simulink model "DuctedFanMolell_V1"  (R2021b)
settings: Solver=VariableStepAuto  StartTime=0.0  StopTime=50.2  MaxStep=0.01  RelTol=1e-3
undefined symbols (not defined in the file or in its folder): SimParam
settings Model: PacingRate=1.300000  VariantFading=off  Creator=tim  LastModifiedBy=tim

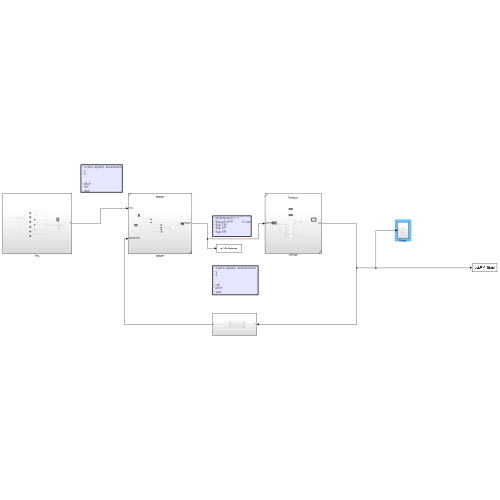
[thumbnail: Simulink's stored preview of the top-level diagram]
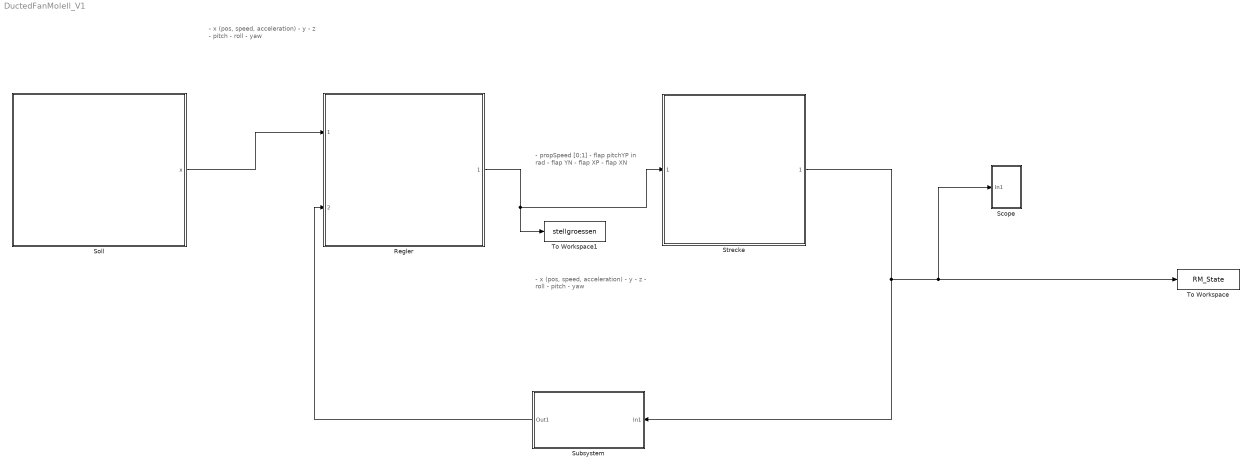
== system DuctedFanMolell_V1 ==
  note: - x (pos, speed, acceleration)
      | - y
      | - z
      |
      |
      | - roll
      | - pitch
      | - yaw
  note: - x (pos, speed, acceleration)
      | - y
      | - z
      |
      |
      | - pitch
      | - roll
      | - yaw
  note: - propSpeed [0;1]
      | - flap pitchYP          in rad
      | - flap YN
      | - flap XP
      | - flap XN
  Regler : Subsystem  VariantControl=Choice  ReferencedSubsystem=Regler
  Scope : Subsystem
  Soll : Subsystem
  Strecke : Subsystem  ReferencedSubsystem=Strecke
  Subsystem : Subsystem
      settings: PortSchema="{\"entries\":[{\"content\":{\"sides\":[{\"content\":{\"connectorIds\":[\"Out1\"]},\"type\":\"ConnectorPlacement.EquallySpacedRectSide\",\"uuid\":\"0b6b1713-0599-4a2b-a6b8-17ca65ceb7bc\"},{\"content\":{\"connectorIds\":[\"In1\"],\"side\":\"RIGHT\"},\"type\":\"ConnectorPlacement.EquallySpacedRectSide\",\"uuid\":\"89969f44-fab1-4e90-b2ff-0e3a2cc6e655\"},{\"content\":{\"connectorIds\":[],\"side\":\"TOP\"},\"type\":\"ConnectorPlacement.EquallySpacedRectSide\",\"uuid\":\"aad73966-e619-409d-ac58-96523cc99cf8\"}]},\"type\":\"ConnectorPlacement.EquallySpacedConnector\",\"uuid\":\"181e3664-8f4e-4946-ae8e-84605a680910\"}],\"packageUris\":[\"http://schema.mathworks.com/mf0/Connector/R2020b\"],\"version\":\"1.0\"}"
  To Workspace : ToWorkspace  VariableName=RM_State  SaveFormat=Timeseries  SampleTime=-1
  To Workspace1 : ToWorkspace  VariableName=stellgroessen  SaveFormat=Timeseries  SampleTime=-1
  wires:
  Soll/1(x) -> Regler/1
  Strecke/1 -> Subsystem/1(In1), Scope/1(In1), To Workspace/1
  Regler/1 -> To Workspace1/1, Strecke/1
  Subsystem/1(Out1) -> Regler/2

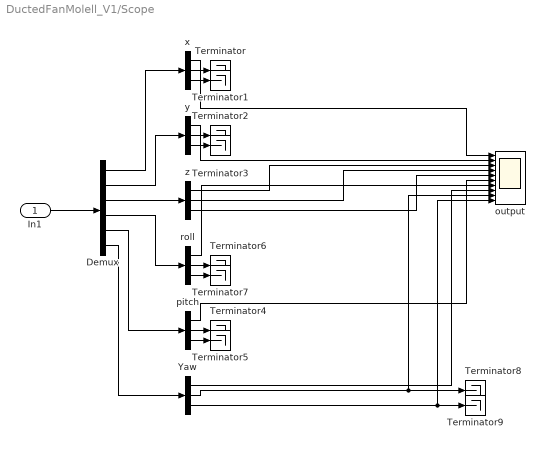
== system DuctedFanMolell_V1/Scope ==
  In1 : Inport
  Demux : Demux  Outputs=[3 3 3 3 3 3]
  Terminator{,1..9} (10 alike) : Terminator
  Yaw : Demux  Outputs=3
  output : Scope  NumInputPorts=10
  pitch : Demux  Outputs=3
  roll : Demux  Outputs=3
  x : Demux  Outputs=3
  y : Demux  Outputs=3
  z : Demux  Outputs=3
  wires:
  Demux/4 -> roll/1
  y/1 -> output/2
  y/2 -> Terminator2/1
  z/3 -> output/5
  Demux/1 -> x/1
  z/2 -> output/4
  roll/2 -> Terminator6/1
  Demux/6 -> Yaw/1
  pitch/3 -> Terminator5/1
  Yaw/2 -> output/9, Terminator8/1
  x/3 -> Terminator1/1
  x/1 -> output/1
  pitch/2 -> Terminator4/1
  Demux/3 -> z/1
  y/3 -> Terminator3/1
  Yaw/3 -> output/10, Terminator9/1
  roll/3 -> Terminator7/1
  pitch/1 -> output/6
  Yaw/1 -> output/8
  In1/1 -> Demux/1
  roll/1 -> output/7
  z/1 -> output/3
  Demux/5 -> pitch/1
  x/2 -> Terminator/1
  Demux/2 -> y/1

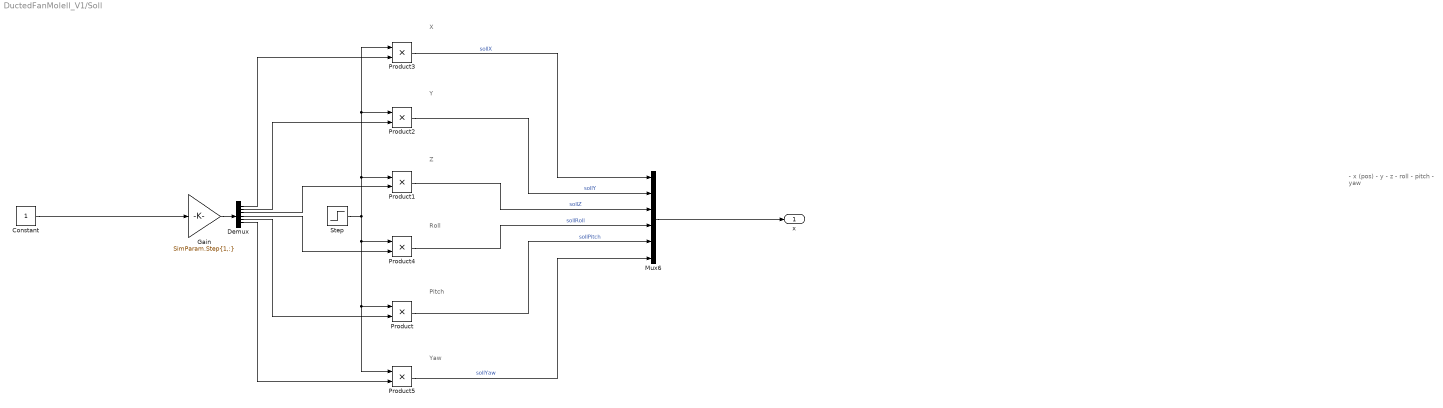
== system DuctedFanMolell_V1/Soll ==
  note: Y
  note: - x (pos)
      | - y
      | - z
      |
      |
      | - roll
      | - pitch
      | - yaw
  note: X
  note: Z
  note: Pitch
  note: Roll
  note: Yaw
  Constant : Constant
  Demux : Demux  Outputs=6
  Gain : Gain  Gain=SimParam.Step{1,:}
  Mux6 : Mux  Inputs=6
  Product{,1..5} (6 alike) : Product
  Step : Step  SampleTime=0
  x : Outport
  wires:
  Product3/1 -> Mux6/1  "sollX"
  Product2/1 -> Mux6/2  "sollY"
  Product1/1 -> Mux6/3  "sollZ"
  Product4/1 -> Mux6/4  "sollRoll"
  Product5/1 -> Mux6/6  "sollYaw"
  Product/1 -> Mux6/5  "sollPitch"
  Mux6/1 -> x/1
  Demux/5 -> Product/2
  Demux/3 -> Product1/2
  Demux/2 -> Product2/2
  Demux/1 -> Product3/2
  Demux/4 -> Product4/2
  Step/1 -> Product5/1, Product/1, Product4/1, Product3/1, Product2/1, Product1/1
  Constant/1 -> Gain/1
  Gain/1 -> Demux/1
  Demux/6 -> Product5/2

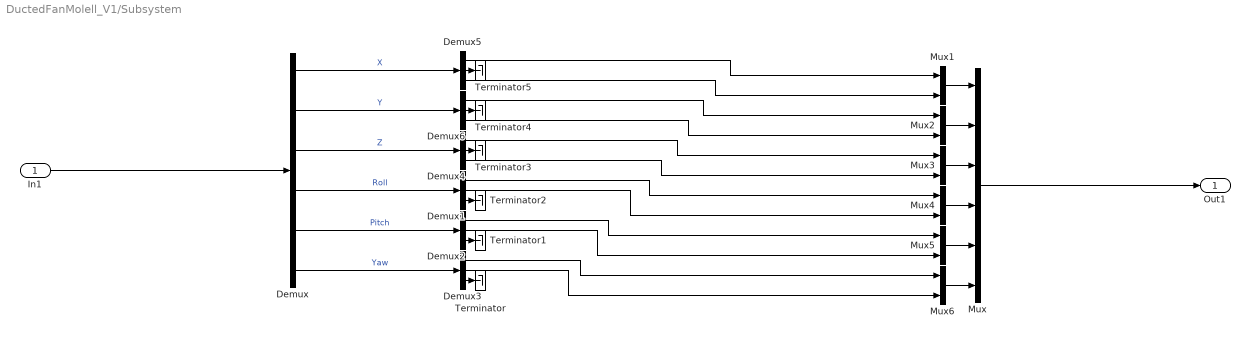
== system DuctedFanMolell_V1/Subsystem ==
  In1 : Inport
  Demux : Demux  Outputs=6
  Demux{1..6} (6 alike) : Demux  Outputs=3
  Mux : Mux  Inputs=6
  Mux{1..6} (6 alike) : Mux  Inputs=2
  Terminator{,1..5} (6 alike) : Terminator
  Out1 : Outport
  wires:
  In1/1 -> Demux/1
  Demux/4 -> Demux1/1  "Roll"
  Demux/3 -> Demux4/1  "Z"
  Demux/2 -> Demux6/1  "Y"
  Demux/1 -> Demux5/1  "X"
  Demux/5 -> Demux2/1  "Pitch"
  Demux/6 -> Demux3/1  "Yaw"
  Demux3/3 -> Terminator/1
  Demux2/3 -> Terminator1/1
  Demux1/3 -> Terminator2/1
  Mux1/1 -> Mux/1
  Mux2/1 -> Mux/2
  Mux3/1 -> Mux/3
  Mux4/1 -> Mux/4
  Mux6/1 -> Mux/6
  Mux5/1 -> Mux/5
  Demux3/2 -> Mux6/2
  Demux3/1 -> Mux6/1
  Demux2/2 -> Mux5/2
  Demux2/1 -> Mux5/1
  Demux1/2 -> Mux4/2
  Demux1/1 -> Mux4/1
  Demux4/1 -> Mux3/1
  Demux4/3 -> Mux3/2
  Demux6/1 -> Mux2/1
  Demux6/3 -> Mux2/2
  Demux5/1 -> Mux1/1
  Demux5/3 -> Mux1/2
  Demux4/2 -> Terminator3/1
  Demux6/2 -> Terminator4/1
  Demux5/2 -> Terminator5/1
  Mux/1 -> Out1/1
